simulink model "flux"  (R2025a)
settings: Solver=VariableStepAuto  StartTime=0.0  StopTime=10.0  RelTol=1e-3
values from neighbouring files (symbols this model uses):
  b1 = 0.0023    [variables.mat]
  b2 = 0.0002    [variables.mat]
  b3 = 0.0001    [variables.mat]
  C = 1    [variables.mat]
  J1 = 0.0025    [variables.mat]
  J2 = 0.0018    [variables.mat]
  J3 = 0.0018    [variables.mat]
  k1 = 2.7    [variables.mat]
  k2 = 2.6    [variables.mat]
settings Model: Creator=jonathantybirk  LastModifiedBy=jonathantybirk

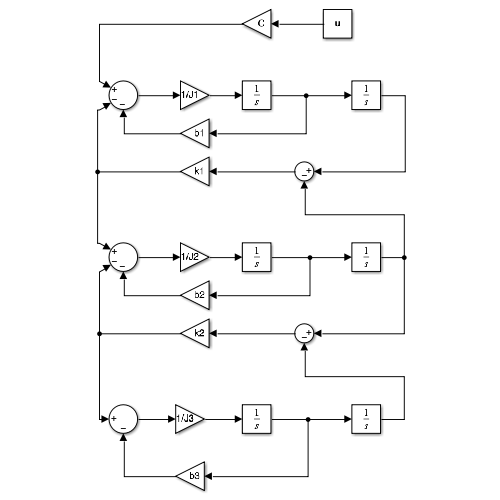
[thumbnail: Simulink's stored preview of the top-level diagram]
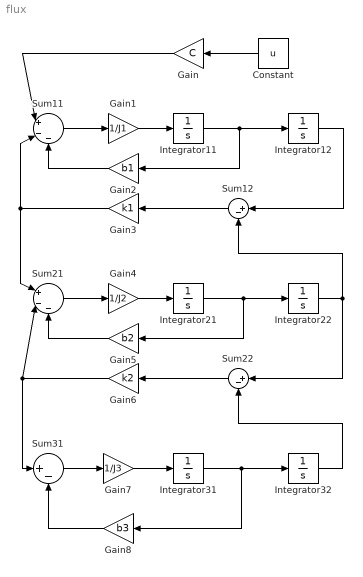
== system flux ==
  Constant : Constant  Value=u
  Gain : Gain  Gain=C
  Gain1 : Gain  Gain=1/J1
  Gain2 : Gain  Gain=b1
  Gain3 : Gain  Gain=k1
  Gain4 : Gain  Gain=1/J2
  Gain5 : Gain  Gain=b2
  Gain6 : Gain  Gain=k2
  Gain7 : Gain  Gain=1/J3
  Gain8 : Gain  Gain=b3
  Integrator{11..12,21..22,31..32} (6 alike) : Integrator
  Sum11 : Sum  Inputs=|+--
  Sum12 : Sum  Inputs=|+-
  Sum21 : Sum  Inputs=|+--
  Sum22 : Sum  Inputs=|+-
  Sum31 : Sum  Inputs=|+-
  wires:
  Gain/1 -> Sum11/1
  Integrator12/1 -> Sum12/1
  Integrator11/1 -> Gain2/1, Integrator12/1
  Gain1/1 -> Integrator11/1
  Sum11/1 -> Gain1/1
  Gain2/1 -> Sum11/3
  Integrator22/1 -> Sum22/1, Sum12/2
  Sum12/1 -> Gain3/1
  Gain3/1 -> Sum21/1, Sum11/2
  Integrator21/1 -> Gain5/1, Integrator22/1
  Gain4/1 -> Integrator21/1
  Sum21/1 -> Gain4/1
  Gain5/1 -> Sum21/3
  Sum22/1 -> Gain6/1
  Gain6/1 -> Sum31/1, Sum21/2
  Integrator31/1 -> Gain8/1, Integrator32/1
  Integrator32/1 -> Sum22/2
  Sum31/1 -> Gain7/1
  Gain7/1 -> Integrator31/1
  Gain8/1 -> Sum31/2
  Constant/1 -> Gain/1
